simulink model "staircase_test"  (Simulink 9.3)
settings: Solver=VariableStepAuto  StartTime=0.0  StopTime=2400  RelTol=1e-3  EnableMultiTasking=on
StartFcn:
  | clear all
libraries: realtime_pacer_lib x1
settings Model: Creator=johnh  LastModifiedBy=hgarnier
settings DataIOCC: SaveFormat=Dataset  SignalLoggingSaveFormat=Dataset
settings DebuggingCC: UnderspecifiedInitializationDetection=Simplified  MergeDetectMultiDrivingBlocksExec=error  FcnCallInpInsideContextMsg=error  PregeneratedLibrarySubsystemCodeDiagnostic=none
settings HardwareCC: ProdBitPerPointer=64  ProdBitPerSizeT=64  ProdBitPerPtrDiffT=64  ProdLargestAtomicFloat=Float  ProdIntDivRoundTo=Zero  ProdEndianess=LittleEndian  ProdWordSize=64  ProdHWDeviceType=Intel->x86-64 (Windows64)
settings ModelReferenceCC: PropagateSignalLabelsOutOfModel=on
settings GRTTargetCC: GeneratePreprocessorConditionals=Disable all  CombineOutputUpdateFcns=on  GRTInterface=off

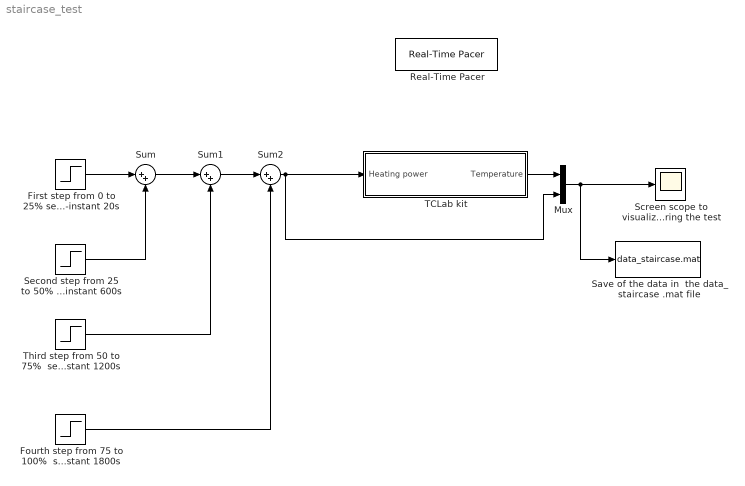
== system staircase_test ==
  " Screen scope to visualize  the signalsduring the test" : Scope
  First step from 0 to 25% sent at time-instant 20s : Step  Time=20  After=25  SampleTime=0
  Fourth step from 75 to 100%  sent at time-instant 1800s : Step  Time=1800  After=25  SampleTime=0
  Mux : Mux  Inputs=2
  Real-Time Pacer : realtime_pacer_lib/Real-Time Pacer  simTimePerRealTime=1
  Save of the data in  the data_staircase .mat file : ToFile  Filename=data_staircase.mat  MatrixName=data0
  Second step from 25 to 50%  sent at time-instant 600s : Step  Time=600  After=25  SampleTime=0
  Sum : Sum  Inputs=|++
  Sum1 : Sum  Inputs=|++
  Sum2 : Sum  Inputs=|++
  TCLab kit : Subsystem
  "Third step from 50 to 75%  sent at time-instant 1200s  " : Step  Time=1200  After=25  SampleTime=0
  wires:
  TCLab kit/1(Temperature) -> Mux/1
  Mux/1 -> Save of the data in  the data_staircase .mat file/1, " Screen scope to visualize  the signalsduring the test"/1
  First step from 0 to 25% sent at time-instant 20s/1 -> Sum/1
  Second step from 25 to 50%  sent at time-instant 600s/1 -> Sum/2
  "Third step from 50 to 75%  sent at time-instant 1200s  "/1 -> Sum1/2
  Fourth step from 75 to 100%  sent at time-instant 1800s/1 -> Sum2/2
  Sum/1 -> Sum1/1
  Sum1/1 -> Sum2/1
  Sum2/1 -> Mux/2, TCLab kit/1(Heating power)

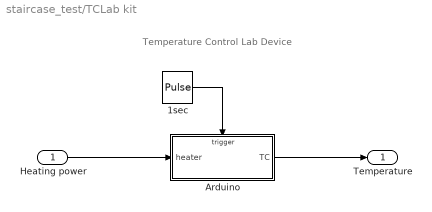
== system staircase_test/TCLab kit ==
  note: Temperature Control Lab Device
  Heating power : Inport
  1sec : DiscretePulseGenerator  PulseType=Time based  Period=1  PulseWidth=50
  Arduino : Subsystem  TreatAsAtomicUnit=on
  Temperature : Outport
  wires:
  1sec/1 -> Arduino/Trigger
  Arduino/1(TC) -> Temperature/1
  Heating power/1 -> Arduino/1(heater)

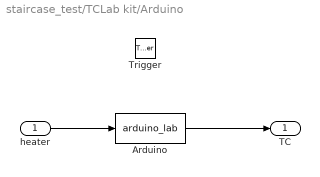
== system staircase_test/TCLab kit/Arduino ==
  heater : Inport
  Trigger : TriggerPort  VariantControl=Variant
  Arduino : MATLABFcn  MATLABFcn=arduino_lab
  TC : Outport  InitialOutput=23
  wires:
  heater/1 -> Arduino/1
  Arduino/1 -> TC/1
